simulink model "IMU_visualiser"  (R2024a)
settings: Solver=FixedStepDiscrete  StartTime=0.0  StopTime=inf  FixedStep=1/fs  RelTol=1e-3
values from neighbouring files (symbols this model uses):
  acc_g = 0.000598550415039    [IMU_visualiser_wrksp.mat]
  fs = 100    [IMU_visualiser_wrksp.mat]
  gyro_g = 0.000133158054504    [IMU_visualiser_wrksp.mat]
undefined symbols (not defined in the file or in its folder): CR, d, f, LF
libraries: dspstat3 x3, sim3dlib x2, matrix_library x2, mspfiltlib x1, robotcorelib x1, simulink x1, instrumentlib x1
settings Model: SimulationMode=accelerator  Creator=DeveloperY  LastModifiedBy=DeveloperY

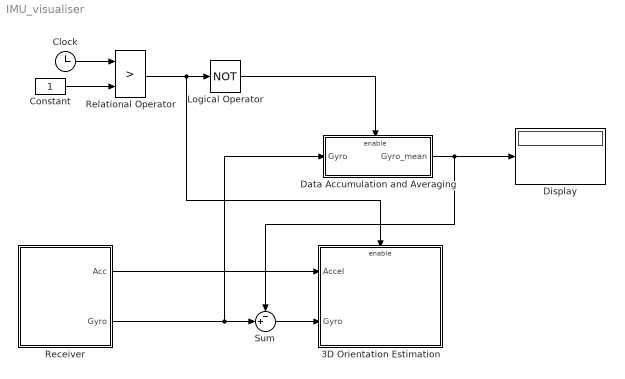
== system IMU_visualiser ==
  3D Orientation Estimation : Subsystem  TreatAsAtomicUnit=on
  Clock : Clock
  Constant : Constant
  Data Accumulation and Averaging : Subsystem  TreatAsAtomicUnit=on
  Display : Display
  Logical Operator : Logic  Operator=NOT  AllPortsSameDT=off  OutDataTypeStr=boolean
  Receiver : Subsystem
  Relational Operator : RelationalOperator  Operator=>  OutDataTypeStr=boolean  RndMeth=Simplest  InputSameDT=off
  Sum : Sum  Inputs=-+|
  wires:
  Receiver/1(Acc) -> 3D Orientation Estimation/1(Accel)
  Receiver/2(Gyro) -> Sum/2, Data Accumulation and Averaging/1(Gyro)
  Clock/1 -> Relational Operator/1
  Relational Operator/1 -> 3D Orientation Estimation/Enable, Logical Operator/1
  Constant/1 -> Relational Operator/2
  Logical Operator/1 -> Data Accumulation and Averaging/Enable
  Data Accumulation and Averaging/1(Gyro_mean) -> Sum/1, Display/1
  Sum/1 -> 3D Orientation Estimation/2(Gyro)

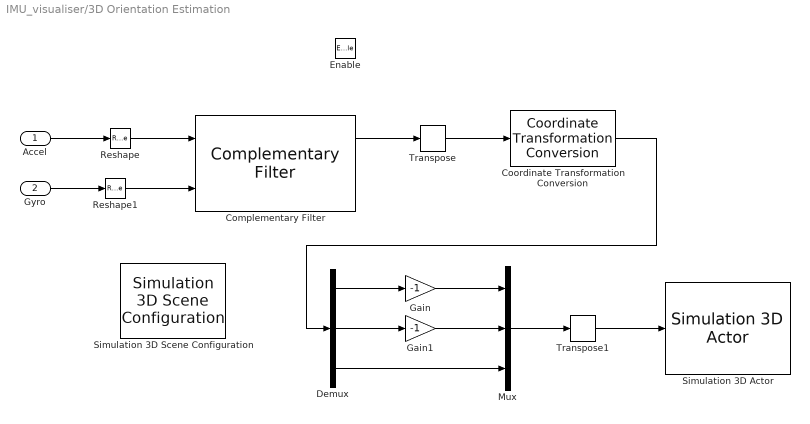
== system IMU_visualiser/3D Orientation Estimation ==
  Accel : Inport
  Gyro : Inport  Port=2
  Enable : EnablePort
  Complementary Filter : mspfiltlib/Complementary Filter  DispRefFrame=ENU  OrientationFormat=quaternion  AccelerometerGain=0.04  HasMagnetometer=off  MagnetometerGain=0.01  SimulateUsing=Code generation
  Coordinate Transformation Conversion : robotcorelib/Coordinate Transformation Conversion  InputRepresentation=Quaternion  InputEulerSequence=ZYX  ShowTrVecInputPort=on  OutputRepresentation=Euler Angles  OutputEulerSequence=XYZ  ShowTrVecOutputPort=on  SimulateUsing=Code generation
      settings: LibrarySourceBlock=uavutilslib/Coordinate Transformation Conversion
  Demux : Demux  Outputs=3
  Gain : Gain  Gain=-1
  Gain1 : Gain  Gain=-1
  Mux : Mux  Inputs=3
  Reshape : Reshape  OutputDimensionality=Customize  OutputDimensions=[1,3]
  Reshape1 : Reshape  OutputDimensionality=Customize  OutputDimensions=[1,3]
  Simulation 3D Actor : sim3dlib/Simulation 3D Actor  Priority=1  ActorName=Sim3dActor1  ParentName=Scene Origin  Operation=Create at setup  InitScriptText=|  SampleTime=-1  Translation=single([0 0 0])  Rotation=single([0 0 0])  Scale=single([1 1 1])  InputsText=Sim3dActor1.Rotation  aMode=5  ActorTag=Sim3dActor1  ActorType=Sim3dActor  ID=1
      | % Reserved keywords:
      | % - Actor : handle to this actor object
      | % - World : handle to the world object
      | 
      | % Examples:
      | 
      | % Create a primitive geometry (optional)
      | %Actor.createShape('box', [30 100 1]);
      | 
      | %Initialize values (optional)
      | Actor.Scale = 0.1;
      | Actor.Color = [1, 1, 1];
  Simulation 3D Scene Configuration : sim3dlib/Simulation 3D Scene Configuration  Priority=0  ProjectFormat=Default Scenes  SceneDesc=Empty scene  ProjectName=C:\Program Files\MATLAB\R2024a\toolbox\shared\sim3d_projects\automotive_project_windows\UE\WindowsNoEditor\VehicleSimulation.exe  ScenePath=/Game/Maps/HwStrght  EnableOpenDRIVE=off  vehTagList={'Custom';'Scene Origin';'Sim3dActor1'}  vehTag=Scene Origin  FreeCameraInitialTranslation=[0, 0, 0]  FreeCameraDefaultInitialTranslation=[-6, 0, 2]  FreeCameraInitialRotation=[0, 0, 0]  FreeCameraDefaultInitialRotation=[0, -15, 0]  OpVisEn=off  Ts=1/fs  EnableWindow=on  EnableRemoteAccess=off  EnableWeather=on  SunAzimuth=30  SunAltitude=90  EnableGeospatialSun=off  Latitude=0  Longitude=0  Date=2023-01-01  Time=10:30:00  GeoTimeZone=-5.0  SunDaylightSaving=off  wind=0  clouds=0.0  EnableVolumetricClouds=off  CloudCoverage=0  CloudAltitude=6  fog=0  rain=0  RaindropsEffect=off  SnowDensity=0  EnableGeospatial=off  UseTrueOrigin=off  OriginHeight=200  OriginLatitude=40.744652  OriginLongitude=-73.988864  MapStyle=Aerial  AdditionalAssetIDs=[]  UseAdvancedSunSky=off  SolarTime=11  TimeZone=-5  Day=21  Month=9  Year=2022  UseDaylightSavingTime=on  DSTStartDay=10  DSTStartMonth=3  DSTEndDay=3  DSTEndMonth=11  DSTSwitchHour=2  sensorTag=MainCamera1  sensorId=1  sensorName=MainCamera1  mountLoc=Origin  offsetFlag=off  tmountOffset=[0, 0, 0]  rmountOffset=[0, 0, 0]  HorizontalResolution=1280  VerticalResolution=720  HorizontalFOV=60  mountPoint=[0 0 0]  mountOrientation=[0 0 0]  aMode=aMode  ID=1  GeoTrigger=Inactive
  Transpose : matrix_library/Transpose
  Transpose1 : matrix_library/Transpose
  wires:
  Transpose/1 -> Coordinate Transformation Conversion/1
  Complementary Filter/1 -> Transpose/1
  Reshape/1 -> Complementary Filter/1
  Transpose1/1 -> Simulation 3D Actor/1
  Reshape1/1 -> Complementary Filter/2
  Accel/1 -> Reshape/1
  Gyro/1 -> Reshape1/1
  Coordinate Transformation Conversion/1 -> Demux/1
  Mux/1 -> Transpose1/1
  Demux/1 -> Gain/1
  Demux/2 -> Gain1/1
  Demux/3 -> Mux/3
  Gain/1 -> Mux/1
  Gain1/1 -> Mux/2

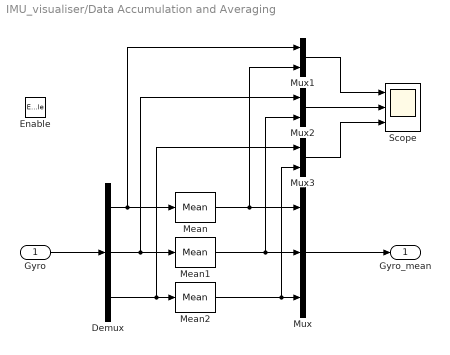
== system IMU_visualiser/Data Accumulation and Averaging ==
  Gyro : Inport
  Enable : EnablePort
  Demux : Demux  Outputs=3
  Mean : dspstat3/Mean  run=on  InputProcessing=Columns as channels (frame based)  reset_popup=None  directionMode=Entire input  dimension=1  roiEnable=off  roiType=Rectangles  roiPortion=Entire ROI  roiOutput=Individual statistics for each ROI  roiFlag=off  roundingMode=Floor  overflowMode=off  outputDataTypeStr=Inherit: Same as accumulator  outputMin=[]  outputMax=[]  outputLastDataTypeStr=Inherit: Same as accumulator
  Mean1 : dspstat3/Mean  run=on  InputProcessing=Columns as channels (frame based)  reset_popup=None  directionMode=Entire input  dimension=1  roiEnable=off  roiType=Rectangles  roiPortion=Entire ROI  roiOutput=Individual statistics for each ROI  roiFlag=off  roundingMode=Floor  overflowMode=off  outputDataTypeStr=Inherit: Same as accumulator  outputMin=[]  outputMax=[]  outputLastDataTypeStr=Inherit: Same as accumulator
  Mean2 : dspstat3/Mean  run=on  InputProcessing=Columns as channels (frame based)  reset_popup=None  directionMode=Entire input  dimension=1  roiEnable=off  roiType=Rectangles  roiPortion=Entire ROI  roiOutput=Individual statistics for each ROI  roiFlag=off  roundingMode=Floor  overflowMode=off  outputDataTypeStr=Inherit: Same as accumulator  outputMin=[]  outputMax=[]  outputLastDataTypeStr=Inherit: Same as accumulator
  Mux : Mux  Inputs=3
  Mux1 : Mux  Inputs=2
  Mux2 : Mux  Inputs=2
  Mux3 : Mux  Inputs=2
  Scope : Scope  NumInputPorts=3
  Gyro_mean : Outport
  wires:
  Gyro/1 -> Demux/1
  Demux/1 -> Mux1/1, Mean/1
  Demux/2 -> Mux2/1, Mean1/1
  Demux/3 -> Mux3/1, Mean2/1
  Mean/1 -> Mux1/2, Mux/1
  Mean1/1 -> Mux2/2, Mux/2
  Mean2/1 -> Mux3/2, Mux/3
  Mux/1 -> Gyro_mean/1
  Mux1/1 -> Scope/1
  Mux2/1 -> Scope/2
  Mux3/1 -> Scope/3

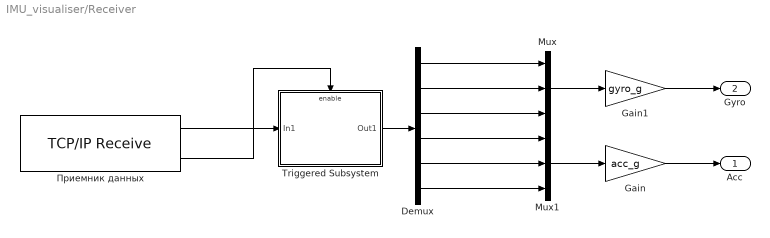
== system IMU_visualiser/Receiver ==
  Demux : Demux  Outputs=6
  Gain : Gain  Gain=acc_g  OutDataTypeStr=single
  Gain1 : Gain  Gain=gyro_g  OutDataTypeStr=single
  Mux : Mux  Inputs=3
  Mux1 : Mux  Inputs=3
  Triggered Subsystem : Subsystem  TreatAsAtomicUnit=on
  Приемник данных : instrumentlib/TCP//IP Receive  Host=192.168.137.73  Port=3333  DataSize=[6]  DataType=int16  ASCIIFormatting=%f,%f,%f,%f,%f,%f,%f,%f,%e,%d  Terminator=CR/LF  CustomTerminator=10  ByteOrder=little-endian  EnableBlockingMode=off  Timeout=10  SampleTime=1/fs  SimulateUsing=Interpreted execution
  Acc : Outport
  Gyro : Outport  Port=2
  wires:
  Приемник данных/1 -> Triggered Subsystem/1(In1)
  Triggered Subsystem/1(Out1) -> Demux/1
  Приемник данных/2 -> Triggered Subsystem/Enable
  Gain1/1 -> Gyro/1
  Mux/1 -> Gain1/1
  Mux1/1 -> Gain/1
  Gain/1 -> Acc/1
  Demux/4 -> Mux1/1
  Demux/5 -> Mux1/2
  Demux/6 -> Mux1/3
  Demux/2 -> Mux/2
  Demux/3 -> Mux/3
  Demux/1 -> Mux/1

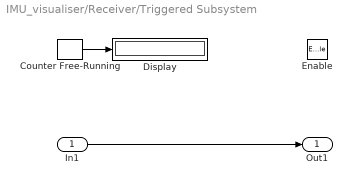
== system IMU_visualiser/Receiver/Triggered Subsystem ==
  In1 : Inport
  Enable : EnablePort
  Counter Free-Running : simulink/Sources/Counter Free-Running  NumBits=16  tsamp=-1
  Display : Display
  Out1 : Outport
  wires:
  In1/1 -> Out1/1
  Counter Free-Running/1 -> Display/1
